simulink model "second"  (Simulink 10.3)
settings: Solver=ode1  StartTime=0.0  StopTime=inf  FixedStep=0.005  RelTol=1e-3  EnableMultiTasking=on
undefined symbols (not defined in the file): HIL
libraries: quarc_library x8, slctrlblks x1, pid_lib x1
settings Model: Creator=rhuq  LastModifiedBy=Rohan  SimulationMode=external  ExtModeTrigDuration=10000
settings Model: SuppressorTable=|
  | <?xml version="1.0" encoding="UTF-8" standalone="yes" ?>
  | <!DOCTYPE boost_serialization>
  | <boost_serialization signature="serialization::archive" version="17">
  | <DiagnosticSuppressor class_id="0" tracking_level="0" version="7">
  | 	<Table class_id="1" tracking_level="0" version="0">
  | 		<count>1</count>
  | 		<bucket_count>8</bucket_count>
  | 		<item_version>0</item_version>
  | 		<item class_id="2" tracking_level="0" version="0">
  | 			<first class_id="3" tracking_level="0" version="7">
  | 				<Source class_id="4" tracking_level="0" version="0">
  | 					<count>1</count>
  | 					<item_version>0</item_version>
  | 					<item>938:869:34</item>
  | 				</Source>
  | 			</first>
  | 			<second class_id="5" tracking_level="0" version="7">
  | 				<SuppressedData class_id="6" tracking_level="0" version="0">
  | 					<count>2</count>
  | 					<bucket_count>8</bucket_count>
  | 					<item_version>0</item_version>
  | 					<item class_id="7" tracking_level="0" version="0">
  | 						<first class_id="8" tracking_level="0" version="7">
  | 							<ID>SimulinkFixedPoint:util:Overflowoccurred</ID>
  | 							<Cause>
  | 								<Source>
  | 									<count>0</count>
  | 									<item_version>0</item_version>
  | 								</Source>
  | 							</Cause>
  | 						</first>
  | 						<second class_id="9" tracking_level="0" version="7">
  | 							<Comment></Comment>
  | 							<User></User>
  | 							<LastModified class_id="10" tracking_level="0" version="0">
  | 								<ptime_date class_id="11" tracking_level="0" version="0">
  | 									<date>20160523</date>
  | 								</ptime_date>
  | 								<ptime_time_duration class_id="12" tracking_level="0" version="1">
  | 									<is_special>0</is_special>
  | 									<time_duration_hours>10</time_duration_hours>
  | 									<time_duration_minutes>57</time_duration_minutes>
  | 									<time_duration_seconds>55</time_duration_seconds>
  | 									<time_duration_fractional_seconds>0</time_duration_fractional_seconds>
  | 								</ptime_time_duration>
  | 							</LastModified>
  | 							<SuppressionType>1</SuppressionType>
  | 						</second>
  | 					</item>
  | 					<item>
  | 						<first>
  | 							<ID>Simulink:DataType:WarningOverFlowDetected</ID>
  | 							<Cause>
  | 								<Source>
  | 									<count>0</count>
  | 									<item_version>0</item_version>
  | 								</Source>
  | 							</Cause>
  | 						</first>
  | 						<second>
  | 							<Comment></Comment>
  | 							<User></User>
  | 							<LastModified>
  | 								<ptime_date>
  | 									<date>20160523</date>
  | 								</ptime_date>
  | 								<ptime_time_duration>
  | 									<is_special>0</is_special>
  | 									<time_duration_hours>10</time_duration_hours>
  | 									<time_duration_minutes>57</time_duration_minutes>
  | 									<time_duration_seconds>55</time_duration_seconds>
  | 									<time_duration_fractional_seconds>0</time_duration_fractional_seconds>
  | 								</ptime_time_duration>
  | 							</LastModified>
  | 							<SuppressionType>1</SuppressionType>
  | 						</second>
  | 					</item>
  | 				</SuppressedData>
  | 			</second>
  | 		</item>
  | 	</Table>
  | </DiagnosticSuppressor>
  | 
  | </boost_serialization>
  | 
  | </boost_serialization>
settings SolverCC: PositivePriorityOrder=on
settings DataIOCC: LimitDataPoints=on
settings OptimizationCC: InitFltsAndDblsToZero=on  LifeSpan=auto
settings DebuggingCC: SaveWithParameterizedLinksMsg=none  SolverPrmCheckMsg=warning  ParameterPrecisionLossMsg=none
settings HardwareCC: ProdLargestAtomicInteger=Long  ProdLargestAtomicFloat=Double  ProdIntDivRoundTo=Zero  ProdEndianess=LittleEndian  ProdHWDeviceType=ARM Compatible->ARM Cortex
settings SFSimCC: SimParseCustomCode=off
settings RTWCC: Description=QUARC Linux Raspberry Pi 3 Target (QBot 2e) Using Toolchain  SystemTargetFile=quarc_linux_pi_3.tlc  TemplateMakefile=quarc_default_tmf  Toolchain=QUARC linux_pi_3 | gmake (64-bit Windows)  BuildConfiguration=Faster Runs
settings STFCustomTargetCC: ConcurrentExecutionCompliant=on  UseToolchainInfoCompliant=on  SystemTargetFile=quarc_linux_pi_3.tlc
settings GRTTargetCC: ParMdlRefBuildCompliant=off  CompOptLevelCompliant=off  MatFileLogging=off  CPPClassGenCompliant=off  ExtMode=on  ExtModeMexFile=quarc_comm  ExtModeMexArgs='-w -d /tmp -uri %u', 'tcpip://192.168.2.30:17002'

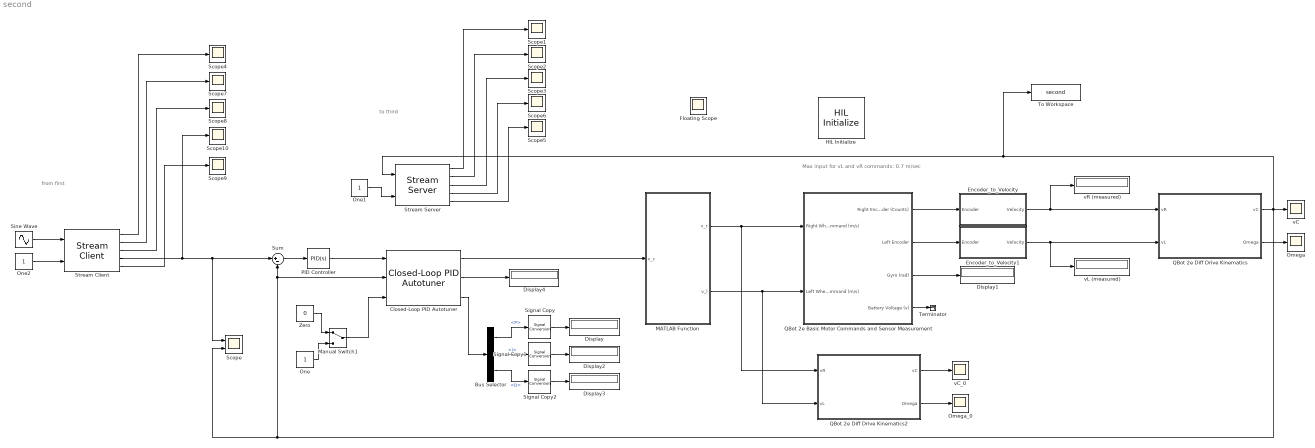
== system second ==
  note: from first
  note: to third
  note: Max input for vL and vR commands: 0.7 m/sec
  Bus Selector : BusSelector  OutputSignals=P,I,D
  Closed-Loop PID Autotuner : slctrlblks/Closed-Loop PID Autotuner  PIDType=PIDF  PIDForm=Parallel  TimeDomain=continuous-time  DiscreteTs=0.1  TuningTs=0.2  UseTuningTs=off  IntegratorFormula=Forward Euler  FilterFormula=Forward Euler  ContinuousTs=0.005  Bandwidth=0.5*6.28  UseExternalWC=off  TargetPM=60  UseExternalPM=off  UseExternalAchievedPM=off  PlantType=Stable  PlantSign=Positive  AmpSine=.3  UseExternalAmpSine=off  UseExternalFRD=off  UseExternalU0=off  UseCompanion=off  NotDeployTuningModule=off  UsePLCCoder=off  OutputMode=control action + perturbation  BlockDataType=double  UseConnectedPID=on  blockpath=[]  tunedP=0  tunedI=0  tunedD=0  tunedN=100  tunedPM=0  EstimationWindowSize=3  UseExternalTuningParams=off  OutputChoice=VariantCandD  SingleMultiRateVariant=SingleSamplingRate
      settings: SourceProductBaseCode=SD
  Display{,1..4} (5 alike) : Display
  Encoder_to_Velocity : Subsystem
  Encoder_to_Velocity1 : Subsystem
  HIL Initialize : quarc_library/Data Acquisition/Generic/Configuration/HIL Initialize  Priority=-99  object_name=HIL-1  board_type=qbot2e  board_number=0  board_options=pwm0_en=1;pwm0_pin=12;pwm1_en=1;pwm1_pin=13;  exclusive=off  active=off  hardware_clocks=[]  clock_modes=[]  initial_clock_frequencies=[]  set_clock_params_at_start=off  set_clock_params_at_switch_in=off  set_clock_frequencies_at_start=off  set_clock_frequencies_at_switch_in=off  analog_input_channels=[0:5]  analog_input_configurations=[]  analog_input_maximums=[16.5 3.3 3.3 3.3 3.3 3.3]  analog_input_minimums=[0 0 0 0 0 0]  set_analog_input_params_at_start=off  set_analog_input_params_at_switch_in=off  analog_output_channels=[]  analog_output_maximums=[]  analog_output_minimums=[]  initial_analog_outputs=[]  final_analog_outputs=[]  watchdog_analog_outputs=[]  set_analog_output_params_at_start=off  set_analog_output_params_at_switch_in=off  set_analog_outputs_at_start=off  set_analog_outputs_at_switch_in=off  set_analog_outputs_at_terminate=off  set_analog_outputs_at_switch_out=off  set_analog_outputs_on_watchdog=off  digital_input_channels=[28:58]  digital_output_channels=[28:31]  digital_output_configuration=[]  initial_digital_outputs=[0]  final_digital_outputs=[0]  watchdog_digital_outputs=[]  set_digital_output_params_at_start=off  set_digital_output_params_at_switch_in=off  set_digital_outputs_at_start=on  set_digital_outputs_at_switch_in=off  set_digital_outputs_at_terminate=on  set_digital_outputs_at_switch_out=off  set_digital_outputs_on_watchdog=off  encoder_channels=[0:1]  quadrature=[4]  encoder_filter_frequency=[]  initial_encoder_counts=[0]  set_encoder_params_at_start=on  set_encoder_params_at_switch_in=off  set_encoder_counts_at_start=on  set_encoder_counts_at_switch_in=off  pwm_channels=[0:1]  pwm_modes=0  pwm_frequency=100e6 / 4095  pwm_configuration=[0]  pwm_alignment=[0]  pwm_polarity=[1]  pwm_leading_deadband=[]  pwm_trailing_deadband=[]  initial_pwm_outputs=[0]  final_pwm_outputs=[0]  watchdog_pwm_outputs=[]  set_pwm_params_at_start=on  set_pwm_params_at_switch_in=off  set_pwm_outputs_at_start=on  set_pwm_outputs_at_switch_in=off  set_pwm_outputs_at_terminate=on  set_pwm_outputs_at_switch_out=off  set_pwm_outputs_on_watchdog=off  other_output_channels=[2000:2001 14000 16000]  initial_other_outputs=[0 0 0 7]  final_other_outputs=[0 0 0 7]  watchdog_other_outputs=[]  set_other_outputs_at_start=on  set_other_outputs_at_switch_in=off  set_other_outputs_at_terminate=on  set_other_outputs_at_switch_out=off  set_other_outputs_on_watchdog=off
  MATLAB Function : MATLAB Function  TreatAsAtomicUnit=on
  Manual Switch1 : ManualSwitch
  Omega : Scope
  Omega_0 : Scope
  One : Constant  OutDataTypeStr=Inherit: Inherit via back propagation
  One1 : Constant  OutDataTypeStr=Inherit: Inherit via back propagation
  One2 : Constant  OutDataTypeStr=Inherit: Inherit via back propagation
  PID Controller : pid_lib/PID Controller  Controller=PID  Form=Parallel  TimeDomain=Continuous-time  UseExternalTs=off  SampleTime=-1  IntegratorMethod=Forward Euler  FilterMethod=Forward Euler  ControllerParametersSource=internal  P=1  I=2  D=0  UseFilter=on  N=0  TunerSelectOption=Frequency Response Based  InitialConditionSource=internal  InitialConditionForIntegrator=0  InitialConditionForFilter=0  DifferentiatorICPrevScaledInput=0  ExternalReset=none  TrackingMode=off  Kt=1  LimitOutput=off  SatLimitsSource=internal  UpperSaturationLimit=inf  LowerSaturationLimit=-inf  LinearizeAsGain=on  AntiWindupMode=none  Kb=1  POutMin=[]  POutMax=[]  IOutMin=[]  IOutMax=[]  DOutMin=[]  DOutMax=[]  NOutMin=[]  NOutMax=[]  SumOutMin=[]  SumOutMax=[]  SaturationOutMin=[]  SaturationOutMax=[]  PParamMin=[]  PParamMax=[]  IParamMin=[]  IParamMax=[]  DParamMin=[]  DParamMax=[]  NParamMin=[]  NParamMax=[]  KbParamMin=[]  KbParamMax=[]  KtParamMin=[]  KtParamMax=[]  KbOutMin=[]  KbOutMax=[]  KtOutMin=[]  KtOutMax=[]  IntegratorOutMin=[]  IntegratorOutMax=[]  FilterOutMin=[]  FilterOutMax=[]  SumI1OutMin=[]  SumI1OutMax=[]  SumI2OutMin=[]  SumI2OutMax=[]  SumI3OutMin=[]  SumI3OutMax=[]  SumI4OutMin=[]  SumI4OutMax=[]  SumDOutMin=[]  SumDOutMax=[]  DifferentiatorOutMin=[]  DifferentiatorOutMax=[]  FilterDiffOutCoefMin=[]  FilterDiffOutCoefMax=[]  ReciprocalOutMin=[]  ReciprocalOutMax=[]  SumDenOutMin=[]  SumDenOutMax=[]  SumNumOutMin=[]  SumNumOutMax=[]  DivideOutMin=[]  DivideOutMax=[]  UdiffTsProdOutMin=[]  UdiffTsProdOutMax=[]  NTsProdOutMin=[]  NTsProdOutMax=[]  UintegralTsProdOutMin=[]  UintegralTsProdOutMax=[]  UngainTsProdOutMin=[]  UngainTsProdOutMax=[]  IntegratorContinuousStateAttributes=''  IntegratorStateMustResolveToSignalObject=off  IntegratorRTWStateStorageClass=Auto  FilterContinuousStateAttributes=''  FilterStateMustResolveToSignalObject=off  FilterRTWStateStorageClass=Auto  ParallelPVariant=InternalParameters  IdealPVariant=Disabled  IVariant=InternalParameters  DVariant=InternalParameters  IntegratorVariant=Continuous  SatVariant=Disabled  AWVariant=Passthrough  PCopyVariant=Disabled  TRVariant=Disabled  FdbkBlocksVariant=Forward  IdealPFdbkVariant=Disabled  SatFdbkVariant=Disabled  DerivativeFilterVariant=ContFilter  NVariant=InternalParameters  NCopyVariant=Disabled  FilterICVariant=InternalICsFilter  IntegratorICVariant=InternalICs  ExternalResetVariant=Disabled  TRSumVariant=Passthrough  SumFdbkVariant=Disabled  SumVariant=Sum_PID  TsampFilterVariant=InternalTs  TsampNgainVariant=Passthrough  TsampIntegralVariant=Passthrough  ExternalSaturationOutDataTypeStr=Inherit: Same as second input
  QBot 2e Basic Motor Commands and Sensor Measurement : Subsystem
  QBot 2e Diff Drive Kinematics : Subsystem
  QBot 2e Diff Drive Kinematics2 : Subsystem
  Scope : Scope  NumInputPorts=2
  Scope{1..10} (10 alike) : Scope
  Signal Copy : SignalConversion  OverrideOpt=off
  Signal Copy1 : SignalConversion  OverrideOpt=off
  Signal Copy2 : SignalConversion  OverrideOpt=off
  Sine Wave : Sin  Amplitude=.3  SampleTime=0
  Stream Client : quarc_library/Communications/Basic/Stream Client  uri_source=Specify via dialog (do not evaluate)  uri=tcpip://192.168.2.32:18000  apply_uri_to_all_configs=on  send_buffer_size=1460  receive_buffer_size=1460  byte_order=little endian (Intel - LSB first)  optimization=Minimum latency  send_options=Send all data  receive_options=Receive all data  default_value=[0]  sample_time=qc_get_step_size  active=off  implementation=Use blocking I/O in a separate thread  send_fifo_size=1000  receive_fifo_size=1000  send_priority=0  receive_priority=0  send_dimensions=off  receive_dimensions=off  max_dimensions=-1  data_type=Inherited via back propagation  type_expr=BusObject
      settings: AttributesFormatString="\"tcpip://192.168.2.32:18000\""
  Stream Server : quarc_library/Communications/Basic/Stream Server  uri_source=Specify via dialog (do not evaluate)  uri=tcpip://localhost:18000  apply_uri_to_all_configs=on  send_buffer_size=1460  receive_buffer_size=1460  byte_order=little endian (Intel - LSB first)  optimization=Minimum latency  send_options=Send all data  receive_options=Receive all data  default_value=[0]  sample_time=qc_get_step_size  active=off  implementation=Use blocking I/O in a separate thread  send_fifo_size=1000  receive_fifo_size=1000  send_priority=0  receive_priority=0  send_dimensions=off  receive_dimensions=off  max_dimensions=-1  data_type=Inherited via back propagation  type_expr=BusObject
      settings: AttributesFormatString="\"tcpip://localhost:18000\""
  Sum : Sum  Inputs=|+-
  Terminator : Terminator
  To Workspace : ToWorkspace  VariableName=second  SaveFormat=Structure With Time  SampleTime=-1
  Zero : Constant  Value=0  OutDataTypeStr=Inherit: Inherit via back propagation
  vC : Scope
  vC_0 : Scope
  vL (measured) : Display
  vR (measured) : Display
  Floating Scope : Scope
  wires:
  QBot 2e Basic Motor Commands and Sensor Measurement/1(Right Encoder (Counts)) -> Encoder_to_Velocity/1(Encoder)
  QBot 2e Basic Motor Commands and Sensor Measurement/2(Left Encoder) -> Encoder_to_Velocity1/1(Encoder)
  QBot 2e Basic Motor Commands and Sensor Measurement/3(Gyro (rad)) -> Display1/1
  Encoder_to_Velocity/1(Velocity) -> vR (measured)/1, QBot 2e Diff Drive Kinematics/1(vR)
  Encoder_to_Velocity1/1(Velocity) -> vL (measured)/1, QBot 2e Diff Drive Kinematics/2(vL)
  QBot 2e Diff Drive Kinematics2/1(vC) -> vC_0/1
  QBot 2e Diff Drive Kinematics2/2(Omega) -> Omega_0/1
  QBot 2e Diff Drive Kinematics/2(Omega) -> Omega/1
  MATLAB Function/1(v_r) -> QBot 2e Diff Drive Kinematics2/1(vR), QBot 2e Basic Motor Commands and Sensor Measurement/1(Right Wheel Command (m/s))
  MATLAB Function/2(v_l) -> QBot 2e Diff Drive Kinematics2/2(vL), QBot 2e Basic Motor Commands and Sensor Measurement/2(Left Wheel Command (m/s))
  QBot 2e Basic Motor Commands and Sensor Measurement/4(Battery Voltage (v)) -> Terminator/1
  QBot 2e Diff Drive Kinematics/1(vC) -> Scope/2, Closed-Loop PID Autotuner/2, Sum/2, To Workspace/1, Stream Server/1, vC/1
  Stream Client/4 -> Scope10/1, Scope/1, Sum/1
  Closed-Loop PID Autotuner/1 -> MATLAB Function/1(v_c)
  Zero/1 -> Manual Switch1/1
  One/1 -> Manual Switch1/2
  Manual Switch1/1 -> Closed-Loop PID Autotuner/3
  Closed-Loop PID Autotuner/3 -> Bus Selector/1
  Bus Selector/1 -> Signal Copy/1  "<P>"
  Bus Selector/2 -> Signal Copy1/1  "<I>"
  Bus Selector/3 -> Signal Copy2/1  "<D>"
  Signal Copy/1 -> Display/1
  Signal Copy1/1 -> Display2/1
  Signal Copy2/1 -> Display3/1
  Closed-Loop PID Autotuner/2 -> Display4/1
  PID Controller/1 -> Closed-Loop PID Autotuner/1
  Sum/1 -> PID Controller/1
  One1/1 -> Stream Server/2
  Stream Server/1 -> Scope1/1
  Stream Server/2 -> Scope2/1
  Stream Server/3 -> Scope3/1
  Stream Server/4 -> Scope6/1
  Stream Server/5 -> Scope5/1
  Stream Client/1 -> Scope4/1
  Stream Client/2 -> Scope7/1
  Stream Client/3 -> Scope8/1
  Stream Client/5 -> Scope9/1
  One2/1 -> Stream Client/2
  Sine Wave/1 -> Stream Client/1

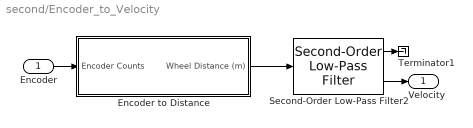
== system second/Encoder_to_Velocity ==
  Encoder : Inport
  Encoder to Distance : Subsystem
  Second-Order Low-Pass Filter2 : quarc_library/Continuous/Second-Order Low-Pass Filter  params_source=Internal (dialog parameters)  input_width=10  input_zeta=1  input_init=0
  Terminator1 : Terminator
  Velocity : Outport
  wires:
  Second-Order Low-Pass Filter2/2 -> Velocity/1
  Encoder/1 -> Encoder to Distance/1(Encoder Counts)
  Encoder to Distance/1(Wheel Distance (m)) -> Second-Order Low-Pass Filter2/1
  Second-Order Low-Pass Filter2/1 -> Terminator1/1

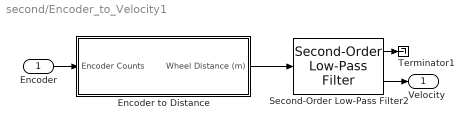
== system second/Encoder_to_Velocity1 ==
  Encoder : Inport
  Encoder to Distance : Subsystem
  Second-Order Low-Pass Filter2 : quarc_library/Continuous/Second-Order Low-Pass Filter  params_source=Internal (dialog parameters)  input_width=10  input_zeta=1  input_init=0
  Terminator1 : Terminator
  Velocity : Outport
  wires:
  Second-Order Low-Pass Filter2/2 -> Velocity/1
  Encoder/1 -> Encoder to Distance/1(Encoder Counts)
  Encoder to Distance/1(Wheel Distance (m)) -> Second-Order Low-Pass Filter2/1
  Second-Order Low-Pass Filter2/1 -> Terminator1/1

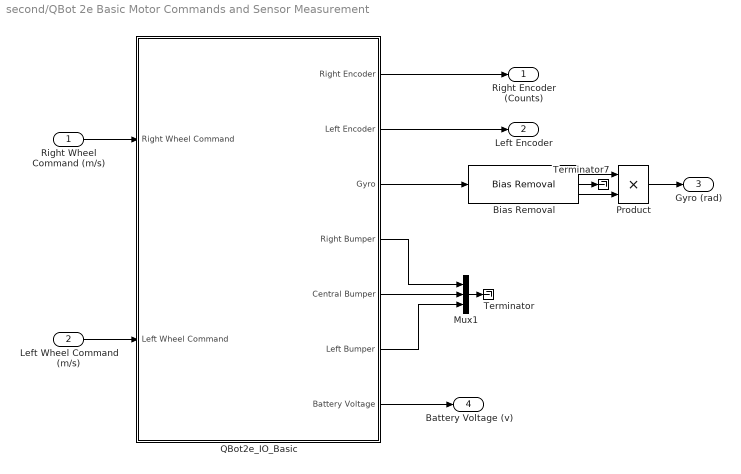
== system second/QBot 2e Basic Motor Commands and Sensor Measurement ==
  Right Wheel Command (m/s) : Inport
  Left Wheel Command (m/s) : Inport  Port=2
  Bias Removal : quarc_library/Discrete/Bias Removal  start_time=3  end_time=4  switch_id=0  sample_time=qc_get_step_size
      settings: SourceProductName=QUARC Targets
  Mux1 : Mux  Inputs=3
  Product : Product  RndMeth=Zero
  QBot2e_IO_Basic : Subsystem
  Terminator : Terminator
  Terminator7 : Terminator
  Right Encoder (Counts) : Outport
  Left Encoder : Outport  Port=2
  Gyro (rad) : Outport  Port=3
  Battery Voltage (v) : Outport  Port=4
  wires:
  QBot2e_IO_Basic/4(Right Bumper) -> Mux1/1
  QBot2e_IO_Basic/5(Central Bumper) -> Mux1/2
  QBot2e_IO_Basic/6(Left Bumper) -> Mux1/3
  Right Wheel Command (m/s)/1 -> QBot2e_IO_Basic/1(Right Wheel Command)
  Left Wheel Command (m/s)/1 -> QBot2e_IO_Basic/2(Left Wheel Command)
  QBot2e_IO_Basic/1(Right Encoder) -> Right Encoder (Counts)/1
  QBot2e_IO_Basic/2(Left Encoder) -> Left Encoder/1
  QBot2e_IO_Basic/7(Battery Voltage) -> Battery Voltage (v)/1
  Bias Removal/2 -> Terminator7/1
  Bias Removal/1 -> Product/1
  Bias Removal/3 -> Product/2
  Product/1 -> Gyro (rad)/1
  QBot2e_IO_Basic/3(Gyro) -> Bias Removal/1
  Mux1/1 -> Terminator/1

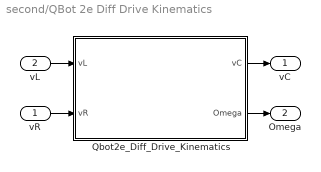
== system second/QBot 2e Diff Drive Kinematics ==
  vR : Inport
  vL : Inport  Port=2
  Qbot2e_Diff_Drive_Kinematics : MATLAB Function  TreatAsAtomicUnit=on
  vC : Outport
  Omega : Outport  Port=2
  wires:
  vL/1 -> Qbot2e_Diff_Drive_Kinematics/1(vL)
  Qbot2e_Diff_Drive_Kinematics/1(vC) -> vC/1
  vR/1 -> Qbot2e_Diff_Drive_Kinematics/2(vR)
  Qbot2e_Diff_Drive_Kinematics/2(Omega) -> Omega/1

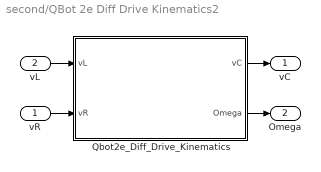
== system second/QBot 2e Diff Drive Kinematics2 ==
  vR : Inport
  vL : Inport  Port=2
  Qbot2e_Diff_Drive_Kinematics : MATLAB Function  TreatAsAtomicUnit=on
  vC : Outport
  Omega : Outport  Port=2
  wires:
  vL/1 -> Qbot2e_Diff_Drive_Kinematics/1(vL)
  Qbot2e_Diff_Drive_Kinematics/1(vC) -> vC/1
  vR/1 -> Qbot2e_Diff_Drive_Kinematics/2(vR)
  Qbot2e_Diff_Drive_Kinematics/2(Omega) -> Omega/1

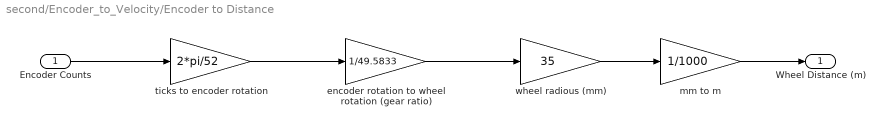
== system second/Encoder_to_Velocity/Encoder to Distance ==
  Encoder Counts : Inport
  " encoder rotation to wheel rotation (gear ratio)" : Gain  Gain=1/49.5833
  mm to m : Gain  Gain=1/1000
  ticks to encoder rotation : Gain  Gain=2*pi/52
  wheel radious (mm) : Gain  Gain=35
  Wheel Distance (m) : Outport
  wires:
  mm to m/1 -> Wheel Distance (m)/1
  wheel radious (mm)/1 -> mm to m/1
  " encoder rotation to wheel rotation (gear ratio)"/1 -> wheel radious (mm)/1
  ticks to encoder rotation/1 -> " encoder rotation to wheel rotation (gear ratio)"/1
  Encoder Counts/1 -> ticks to encoder rotation/1

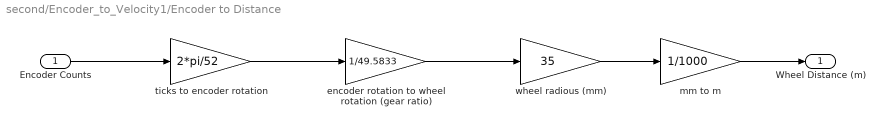
== system second/Encoder_to_Velocity1/Encoder to Distance ==
  Encoder Counts : Inport
  " encoder rotation to wheel rotation (gear ratio)" : Gain  Gain=1/49.5833
  mm to m : Gain  Gain=1/1000
  ticks to encoder rotation : Gain  Gain=2*pi/52
  wheel radious (mm) : Gain  Gain=35
  Wheel Distance (m) : Outport
  wires:
  mm to m/1 -> Wheel Distance (m)/1
  wheel radious (mm)/1 -> mm to m/1
  " encoder rotation to wheel rotation (gear ratio)"/1 -> wheel radious (mm)/1
  ticks to encoder rotation/1 -> " encoder rotation to wheel rotation (gear ratio)"/1
  Encoder Counts/1 -> ticks to encoder rotation/1

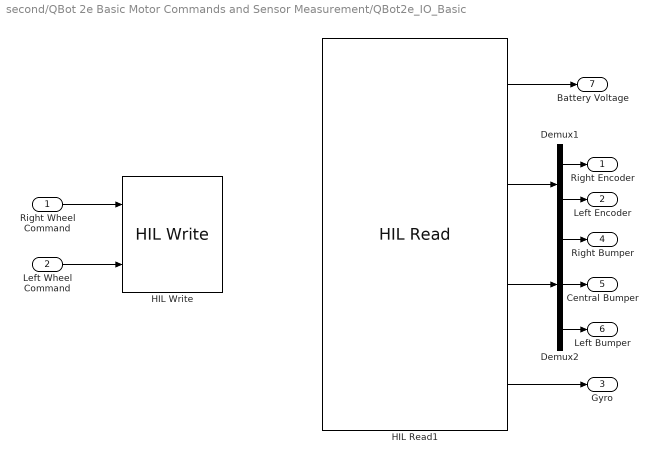
== system second/QBot 2e Basic Motor Commands and Sensor Measurement/QBot2e_IO_Basic ==
  Right Wheel Command : Inport
  Left Wheel Command : Inport  Port=2
  Demux1 : Demux  Outputs=2
  Demux2 : Demux  Outputs=3
  HIL Read1 : quarc_library/Data Acquisition/Generic/Immediate I//O/HIL Read  object_name=HIL-1  analog_channels=[0]  encoder_channels=[0:1]  digital_channels=[28:30]  other_channels=[1002]  sample_time=qc_get_step_size  active=on  vector_output=on  data_type_mode=Inherit via back propagation  encoder_data_type=double  digital_data_type=boolean
  HIL Write : quarc_library/Data Acquisition/Generic/Immediate I//O/HIL Write  object_name=HIL-1  analog_channels=[]  pwm_channels=[]  digital_channels=[]  other_channels=[2000:2001]  sample_time=-1  active=on  vector_input=off
  Right Encoder : Outport
  Left Encoder : Outport  Port=2
  Gyro : Outport  Port=3
  Right Bumper : Outport  Port=4
  Central Bumper : Outport  Port=5
  Left Bumper : Outport  Port=6
  Battery Voltage : Outport  Port=7
  wires:
  HIL Read1/1 -> Battery Voltage/1
  HIL Read1/3 -> Demux2/1
  HIL Read1/4 -> Gyro/1
  Demux1/1 -> Right Encoder/1
  Demux1/2 -> Left Encoder/1
  Right Wheel Command/1 -> HIL Write/1
  Left Wheel Command/1 -> HIL Write/2
  HIL Read1/2 -> Demux1/1
  Demux2/1 -> Right Bumper/1
  Demux2/2 -> Central Bumper/1
  Demux2/3 -> Left Bumper/1

== matlab function QBot 2e Diff Drive Kinematics2/Qbot2e_Diff_Drive_Kinematics ==
  data: vL input double; vC output double; vR input double; Omega output double
function [vC,Omega] = fcn(vL,vR)
%#codegen

d= 0.235;

vC=0.5*(vL+vR);
Omega=(1/d)*(vR-vL);

== matlab function QBot 2e Diff Drive Kinematics/Qbot2e_Diff_Drive_Kinematics ==
  data: vL input double; vC output double; vR input double; Omega output double
function [vC,Omega] = fcn(vL,vR)
%#codegen

d= 0.235;

vC=0.5*(vL+vR);
Omega=(1/d)*(vR-vL);

== matlab function MATLAB Function ==
  data: v_c input double; v_r output double; v_l output double
function [v_r, v_l] = inverse_kinematics(v_c)

v_r = v_c;
v_l = v_c;
